simulink model "gm_ESP8266_Config"  (R2015b)
settings: Solver=VariableStepAuto  StartTime=0.0  StopTime=10.0  RelTol=1e-3
settings Model: Creator=Administrator  LastModifiedBy=Administrator
settings OptimizationCC: BlockReduction=off  ConditionallyExecuteInputs=off
settings DebuggingCC: InheritedTsInSrcMsg=none

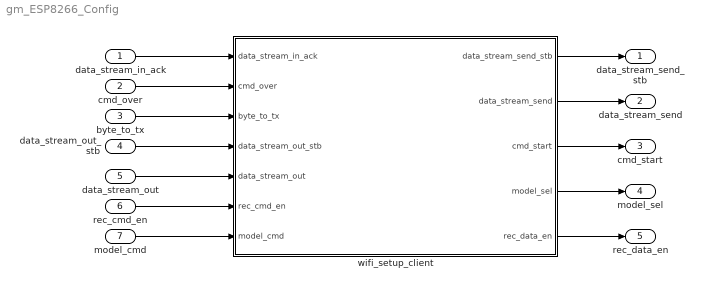
== system gm_ESP8266_Config ==
  data_stream_in_ack : Inport  SampleTime=0
  cmd_over : Inport  Port=2  SampleTime=0
  byte_to_tx : Inport  Port=3  SampleTime=0
  data_stream_out_stb : Inport  Port=4  SampleTime=0
  data_stream_out : Inport  Port=5  SampleTime=0
  rec_cmd_en : Inport  Port=6  SampleTime=0
  model_cmd : Inport  Port=7  SampleTime=0
  "wifi_setup_client " : Subsystem
  data_stream_send_stb : Outport
  data_stream_send : Outport  Port=2
  cmd_start : Outport  Port=3
  model_sel : Outport  Port=4
  rec_data_en : Outport  Port=5
  wires:
  data_stream_in_ack/1 -> "wifi_setup_client "/1(data_stream_in_ack)
  cmd_over/1 -> "wifi_setup_client "/2(cmd_over)
  byte_to_tx/1 -> "wifi_setup_client "/3(byte_to_tx)
  data_stream_out_stb/1 -> "wifi_setup_client "/4(data_stream_out_stb)
  data_stream_out/1 -> "wifi_setup_client "/5(data_stream_out)
  rec_cmd_en/1 -> "wifi_setup_client "/6(rec_cmd_en)
  model_cmd/1 -> "wifi_setup_client "/7(model_cmd)
  "wifi_setup_client "/1(data_stream_send_stb) -> data_stream_send_stb/1
  "wifi_setup_client "/2(data_stream_send) -> data_stream_send/1
  "wifi_setup_client "/3(cmd_start) -> cmd_start/1
  "wifi_setup_client "/4(model_sel) -> model_sel/1
  "wifi_setup_client "/5(rec_data_en) -> rec_data_en/1

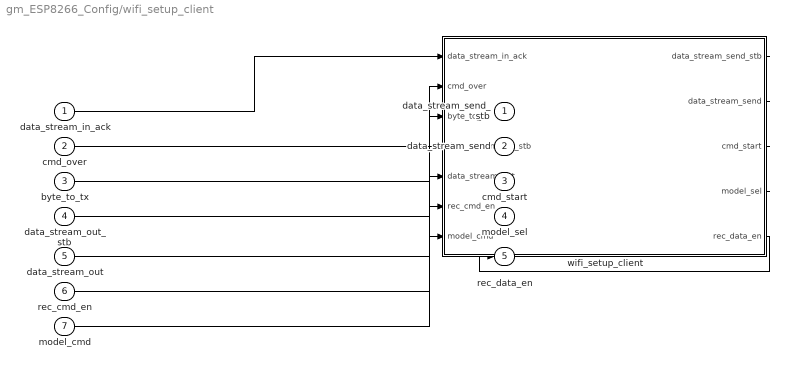
== system gm_ESP8266_Config/wifi_setup_client  ==
  data_stream_in_ack : Inport  SampleTime=0
  cmd_over : Inport  Port=2  SampleTime=0
  byte_to_tx : Inport  Port=3  SampleTime=0
  data_stream_out_stb : Inport  Port=4  SampleTime=0
  data_stream_out : Inport  Port=5  SampleTime=0
  rec_cmd_en : Inport  Port=6  SampleTime=0
  model_cmd : Inport  Port=7  SampleTime=0
  "wifi_setup_client " : Stateflow chart  TreatAsAtomicUnit=on
  data_stream_send_stb : Outport
  data_stream_send : Outport  Port=2
  cmd_start : Outport  Port=3
  model_sel : Outport  Port=4
  rec_data_en : Outport  Port=5
  wires:
  data_stream_in_ack/1 -> "wifi_setup_client "/1(data_stream_in_ack)
  cmd_over/1 -> "wifi_setup_client "/2(cmd_over)
  byte_to_tx/1 -> "wifi_setup_client "/3(byte_to_tx)
  data_stream_out_stb/1 -> "wifi_setup_client "/4(data_stream_out_stb)
  data_stream_out/1 -> "wifi_setup_client "/5(data_stream_out)
  rec_cmd_en/1 -> "wifi_setup_client "/6(rec_cmd_en)
  model_cmd/1 -> "wifi_setup_client "/7(model_cmd)
  "wifi_setup_client "/1(data_stream_send_stb) -> data_stream_send_stb/1
  "wifi_setup_client "/2(data_stream_send) -> data_stream_send/1
  "wifi_setup_client "/3(cmd_start) -> cmd_start/1
  "wifi_setup_client "/4(model_sel) -> model_sel/1
  "wifi_setup_client "/5(rec_data_en) -> rec_data_en/1

== stateflow chart gm_ESP8266_Config/wifi_setup_client /wifi_setup_client  ==
  settings: executeAtInitialization=1
  state initial
    entry:
    data_stream_send_stb=0;
    data_stream_send=0;
    cmd_start=0;
    rec_data_en=0;
    model_sel=0;
    cnt_wait=0;
    cnt_halt=0;
  state Tran_Enter_1
    entry: data_stream_send_stb=1;
    data_stream_send=10;%/n
  state Tran_T
    entry: data_stream_send_stb=1;
    data_stream_send=84;%T
  state Tran_Enter
    entry: data_stream_send_stb=1;
    data_stream_send=13;%/r
  state Tran_A
    entry: data_stream_send_stb=1;
    data_stream_send=65;%A
  state send_finish
    entry: data_stream_send_stb=0;
    data_stream_send=0;
  state wait_cnt1
    entry: cnt_wait=cnt_wait+1;
  state wait_cmd
    entry: cmd_start=1;
    data_stream_send_stb=1;
    data_stream_send=byte_to_tx;
  state send_cmd1
    entry: cmd_start=1;
    data_stream_send_stb=0;
    data_stream_send=byte_to_tx;
  state send_cmd2
    entry: cmd_start=1;
    data_stream_send_stb=1;
    data_stream_send=byte_to_tx;
  state device_OK
    entry: model_sel=model_sel+1;
    cnt_wait=0;
  state send_cmd_over
    entry: cmd_start=0;
    data_stream_send_stb=0;
    data_stream_send=0;
  state Tran1_Enter
    entry: data_stream_send_stb=1;
    data_stream_send=13;%/r
  state Tran1_Enter_1
    entry: data_stream_send_stb=1;
    data_stream_send=10;%/n
  state send_finish1
    entry: data_stream_send_stb=0;
    data_stream_send=0;
  state send_data2
    entry:
    cmd_start=1;
    data_stream_send_stb=1;
    data_stream_send=byte_to_tx;
  state send_data1
    entry:
    cmd_start=1;
    data_stream_send_stb=0;
    data_stream_send=byte_to_tx;
    cnt_halt=0;
  state wait_data
    entry:
    cmd_start=1;
    data_stream_send_stb=1;
    data_stream_send=byte_to_tx;
  state device_config_OK
    entry: model_sel=7;
    %begin sending data
  state send_data_over
    entry:
    cmd_start=0;
    data_stream_send_stb=0;
    data_stream_send=0;
  state send_finish2
    entry: data_stream_send_stb=0;
    data_stream_send=0;
    %After finish sending, I can still get
    % response OK
    cnt_halt=cnt_halt+1;
  state Tran2_Enter
    entry: data_stream_send_stb=1;
    data_stream_send=13;%/r
  state Tran2_Enter_1
    entry: data_stream_send_stb=1;
    data_stream_send=10;%/n
  state wait_client_rec_R
    rec_data_en=1;
    cnt_halt=0;
  state wait_client_rec_C
    entry:
    data_stream_send_stb=0;
    data_stream_send=0;
    cnt_halt=cnt_halt+1;
  state pre_rec_data
  state model_reselect
    entry:
    cnt_halt=0;
    model_sel=5;
  state wait_port
    rec_data_en=0;
    cnt_halt=cnt_halt+1;
  state rec_data
    cnt_halt=cnt_halt+1;
  state restart
    entry:
    cnt_halt=0;
  state send_finish3
    entry:
    data_stream_send_stb=0;
    data_stream_send=0;
    model_sel=0;
  state send_cmd3
    entry: cmd_start=1;
    data_stream_send_stb=0;
    data_stream_send=byte_to_tx;
    cnt_halt=0;
  state wait_cmd1
    entry: cmd_start=1;
    data_stream_send_stb=1;
    data_stream_send=byte_to_tx;
  state send_cmd4
    entry: cmd_start=1;
    data_stream_send_stb=1;
    data_stream_send=byte_to_tx;
  state send_cmd_over1
    entry: cmd_start=0;
    data_stream_send_stb=0;
    data_stream_send=0;
  state Tran3_Enter
    entry: data_stream_send_stb=1;
    data_stream_send=13;%/r
  state Tran3_Enter_1
    entry: data_stream_send_stb=1;
    data_stream_send=10;%/n
  state model_sel_rst
    entry:cnt_halt=0;
    model_sel=9;
  (default) -> initial
  (junction 219) -> initial
  (junction 179) -> (junction 219)
  initial -> Tran_A
  (junction 22) -> Tran_Enter_1 [order 2] : [data_stream_in_ack==0]
  Tran_Enter -> (junction 19)
  (junction 19) -> Tran_Enter_1 [order 1] : [data_stream_in_ack==1]
  Tran_A -> (junction 6)
  (junction 6) -> Tran_T [order 2] : [data_stream_in_ack==1]
  Tran_T -> (junction 14)
  (junction 14) -> Tran_Enter [order 1] : [data_stream_in_ack==1]
  (junction 19) -> Tran_Enter [order 2] : [data_stream_in_ack==0]
  (junction 14) -> Tran_T [order 2] : [data_stream_in_ack==0]
  (junction 6) -> Tran_A [order 1] : [data_stream_in_ack==0]
  Tran_Enter_1 -> (junction 22)
  (junction 29) -> Tran_A [order 1] : [model_cmd~=1]
  (junction 22) -> send_finish [order 1] : [data_stream_in_ack==1]
  (junction 26) -> (junction 29) [order 2] : [rec_cmd_en==1]
  send_finish -> (junction 26)
  (junction 26) -> send_finish [order 1] : [rec_cmd_en==0]
  (junction 29) -> wait_cnt1 [order 2] : [model_cmd==1]
  (junction 132) -> wait_cnt1
  (junction 131) -> (junction 132)
  (junction 34) -> wait_cnt1 [order 1] : [cnt_wait<10000000]%0.05s
  wait_cnt1 -> (junction 34)
  (junction 77) -> wait_cnt1
  (junction 34) -> (junction 37) [order 2] : [cnt_wait>=10000000]
  (junction 45) -> send_cmd2 [order 1] : [data_stream_in_ack==0]
  send_cmd1 -> send_cmd2
  device_OK -> send_cmd1
  (junction 37) -> device_OK [order 1] : [model_sel~=6]
  send_cmd2 -> (junction 45)
  (junction 45) -> wait_cmd [order 2] : [data_stream_in_ack==1]
  (junction 37) -> device_config_OK [order 2] : [model_sel==6]
  (junction 73) -> send_cmd1 [order 1] : [model_cmd~=1]%This cmd does not config sucessfully
  (junction 50) -> send_cmd1 [order 2] : [cmd_over==0]
  wait_cmd -> (junction 50)
  (junction 50) -> send_cmd_over [order 1] : [cmd_over==1]
  send_cmd_over -> Tran1_Enter
  Tran1_Enter -> (junction 60)
  (junction 60) -> Tran1_Enter_1 [order 1] : [data_stream_in_ack==1]
  (junction 66) -> Tran1_Enter_1 [order 2] : [data_stream_in_ack==0]
  (junction 60) -> Tran1_Enter [order 2] : [data_stream_in_ack==0]
  Tran1_Enter_1 -> (junction 66)
  (junction 66) -> send_finish1 [order 1] : [data_stream_in_ack==1]
  (junction 73) -> (junction 77) [order 2] : [model_cmd==1]
  (junction 70) -> (junction 73) [order 2] : [rec_cmd_en==1]
  send_finish1 -> (junction 70)
  (junction 70) -> send_finish1 [order 1] : [rec_cmd_en==0]
  (junction 105) -> send_data2 [order 1] : [data_stream_in_ack==0]
  send_data1 -> send_data2
  send_data2 -> (junction 105)
  (junction 105) -> wait_data [order 2] : [data_stream_in_ack==1]
  device_config_OK -> send_data1
  wait_data -> (junction 111)
  (junction 111) -> send_data2 [order 2] : [cmd_over==0]
  (junction 111) -> send_data_over [order 1] : [cmd_over==1]
  (junction 119) -> Tran2_Enter_1 [order 2] : [data_stream_in_ack==0]
  (junction 118) -> Tran2_Enter [order 2] : [data_stream_in_ack==0]
  (junction 182) -> send_finish2 [order 1] : [cnt_halt<=1000000000]%10sec
  Tran2_Enter_1 -> (junction 119)
  (junction 119) -> send_finish2 [order 1] : [data_stream_in_ack==1]
  send_data_over -> Tran2_Enter
  Tran2_Enter -> (junction 118)
  (junction 118) -> Tran2_Enter_1 [order 1] : [data_stream_in_ack==1]
  send_finish2 -> (junction 155)
  (junction 166) -> pre_rec_data [order 1] : [data_stream_out_stb==0]
  (junction 170) -> rec_data [order 1] : [cnt_halt<8]
  wait_client_rec_R -> pre_rec_data
  (junction 170) -> wait_port [order 2] : [cnt_halt==8]{cnt_halt=0;}
  rec_data -> (junction 170)
  (junction 166) -> rec_data [order 2] : [data_stream_out_stb==1]
  pre_rec_data -> (junction 166)
  (junction 159) -> wait_client_rec_R [order 1] : [(data_stream_out_stb==1) && (data_stream_out==82)]
      | %rec of R
  wait_client_rec_C -> (junction 159)
  (junction 155) -> wait_client_rec_C [order 1] : [(data_stream_out_stb==1) && (data_stream_out==67)]
      | %rec of C
  model_reselect -> (junction 131)
  (junction 120) -> model_reselect [order 2] : [cnt_halt>10000000]
  wait_port -> (junction 120)
  (junction 120) -> wait_port [order 1] : [cnt_halt<=10000000]%0.1s
  (junction 159) -> (junction 221) [order 2] : [(data_stream_out_stb~=1) || (data_stream_out~=82)]
  (junction 155) -> (junction 182) [order 2] : [(data_stream_out_stb~=1) || (data_stream_out~=67)]
      | % not rec C
  (junction 221) -> wait_client_rec_C [order 1] : [cnt_halt<=1000000000]%10sec
  (junction 182) -> restart [order 2] : [cnt_halt>1000000000]%10sec
  (junction 221) -> restart [order 2] : [cnt_halt>1000000000]%10sec
  restart -> model_sel_rst
  (junction 190) -> send_cmd4 [order 1] : [data_stream_in_ack==0]
  (junction 209) -> Tran3_Enter [order 1] : [data_stream_in_ack==0]
  (junction 215) -> Tran3_Enter_1 [order 1] : [data_stream_in_ack==0]
  send_cmd_over1 -> Tran3_Enter
  model_sel_rst -> send_cmd3
  send_finish3 -> (junction 179)
  (junction 209) -> Tran3_Enter_1 [order 2] : [data_stream_in_ack==1]
  Tran3_Enter -> (junction 209)
  (junction 195) -> send_cmd_over1 [order 2] : [cmd_over==1]
  wait_cmd1 -> (junction 195)
  (junction 190) -> wait_cmd1 [order 2] : [data_stream_in_ack==1]
  send_cmd4 -> (junction 190)
  send_cmd3 -> send_cmd4
  (junction 215) -> send_finish3 [order 2] : [data_stream_in_ack==1]
  Tran3_Enter_1 -> (junction 215)
  (junction 195) -> send_cmd3 [order 1] : [cmd_over==0]
  data: data_stream_in_ack input boolean; cmd_over input boolean; byte_to_tx input uint8; data_stream_out_stb input boolean; data_stream_out input uint8; rec_cmd_en input boolean; model_cmd input fixdt(0,4,0); cnt_wait local uint32; data_stream_send_stb output boolean; data_stream_send output uint8; cmd_start output boolean; model_sel output fixdt(0,4,0); rec_data_en output boolean; cnt_halt local int32
